simulink model "MagLev"  (R2023a)
settings: Solver=ode4  StartTime=0.0  StopTime=20  RelTol=1e-3
settings Model: Creator=Pc  LastModifiedBy=mluser
settings SolverCC: AlgebraicLoopSolver=TrustRegion
settings DebuggingCC: SolverPrmCheckMsg=error  UnconnectedInputMsg=warning  UnconnectedOutputMsg=warning  UnconnectedLineMsg=warning
settings ModelReferenceCC: EnableRefExpFcnMdlSchedulingChecks=on

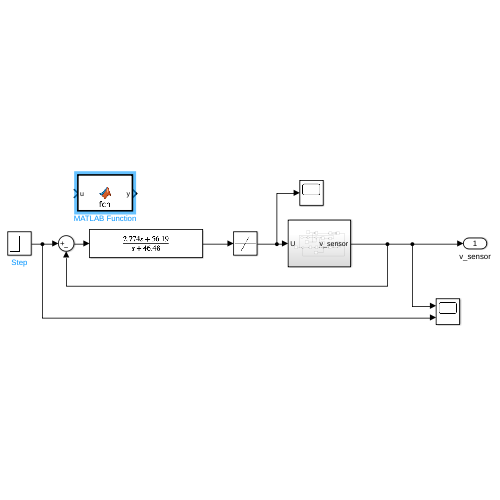
[thumbnail: Simulink's stored preview of the top-level diagram]
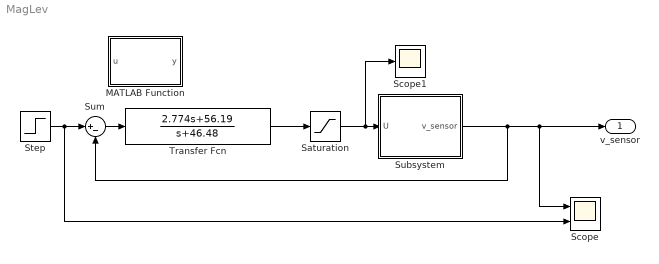
== system MagLev ==
  MATLAB Function : MATLAB Function  TreatAsAtomicUnit=on
  Saturation : Saturate  UpperLimit=5  LowerLimit=-5
  Scope : Scope  NumInputPorts=2
  Scope1 : Scope
  Step : Step  SampleTime=0
  Subsystem : Subsystem
  Sum : Sum  Inputs=|+-
  Transfer Fcn : TransferFcn  Numerator=[2.774 56.19]  Denominator=[1 46.48]
  v_sensor : Outport
  wires:
  Subsystem/1(v_sensor) -> Sum/2, Scope/1, v_sensor/1
  Transfer Fcn/1 -> Saturation/1
  Sum/1 -> Transfer Fcn/1
  Step/1 -> Sum/1, Scope/2
  Saturation/1 -> Scope1/1, Subsystem/1(U)

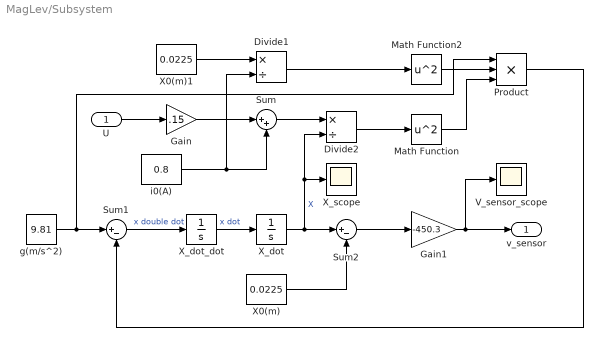
== system MagLev/Subsystem ==
  U : Inport
  Divide1 : Product  Inputs=*/
  Divide2 : Product  Inputs=*/
  Gain : Gain  Gain=.15
  Gain1 : Gain  Gain=-450.3
  Math Function : Math  Operator=square
  Math Function2 : Math  Operator=square
  Product : Product  Inputs=3
  Sum : Sum  Inputs=|++
  Sum1 : Sum  Inputs=|+-
  Sum2 : Sum  Inputs=|+-
  V_sensor_scope : Scope
  X0(m) : Constant  Value=0.0225
  X0(m)1 : Constant  Value=0.0225
  X_dot : Integrator  InitialCondition=0.018  UpperSaturationLimit=.027  LowerSaturationLimit=0.018
  X_dot_dot : Integrator
  X_scope : Scope
  g(m/s^2) : Constant  Value=9.81
  i0(A) : Constant  Value=0.8
  v_sensor : Outport
  wires:
  X0(m)/1 -> Sum2/2
  X_dot/1 -> Divide2/2, X_scope/1, Sum2/1  "X"
  U/1 -> Gain/1
  X_dot_dot/1 -> X_dot/1  "x dot"
  Product/1 -> Sum1/2
  X0(m)1/1 -> Divide1/1
  Divide1/1 -> Math Function2/1
  Divide2/1 -> Math Function/1
  Math Function2/1 -> Product/2
  i0(A)/1 -> Sum/2, Divide1/2
  g(m/s^2)/1 -> Sum1/1, Product/1
  Sum1/1 -> X_dot_dot/1  "x double dot"
  Gain/1 -> Sum/1
  Sum2/1 -> Gain1/1
  Math Function/1 -> Product/3
  Gain1/1 -> v_sensor/1, V_sensor_scope/1
  Sum/1 -> Divide2/1

== matlab function MagLev/MATLAB Function ==
  data: u input; y output
function y = fcn(u)
persistent e_prev;
persistent u_prev;
if(isempty(e_prev)&&isempty(u_prev))
    e_prev =0;
    u_prev =0;
end

Ts = 0.001
a = ;
b = ;
k = ;


end
